simulink model "q_srv02_pos"  (Simulink 6.6)
settings: Solver=ode1  StartTime=0.0  StopTime=inf  FixedStep=0.001  RelTol=1e-3  AbsTol=1e-6
values from neighbouring files (symbols this model uses):
  K_AMP = 1    [setup_srv02_exp02_pos.m]
  ki = -( -AmpMax + kp * e_ss ) / ti / e_ss    [d_i_design.m]    (also in setup_srv02_exp02_pos.m = 0)
  kp = wn^2/K*tau    [d_pv_design.m]    (also in setup_srv02_exp02_pos.m = 0)
  kv = (-1+2*zeta*wn*tau)/K    [d_pv_design.m]    (also in setup_srv02_exp02_pos.m = 0)
  VMAX_DAC = 10    [setup_srv02_exp02_pos.m]
  wcf = 2 * pi * 50.0    (= 314.159265359)    [setup_srv02_exp02_pos.m]
  wcf_e = 2 * pi * 50.0    (= 314.159265359)    [setup_srv02_exp02_pos.m]
  zetaf = 0.9    [setup_srv02_exp02_pos.m]
  zetaf_e = 0.9    [setup_srv02_exp02_pos.m]
undefined symbols (not defined in the file or in its folder): HIL, K_ENC, K_POT, K_TACH, qc_get_step_size, VMAX_AMP
libraries: quarc_library x6
settings Model: Creator=MLevis  LastModifiedBy=MLevis  SimulationMode=external  ExtModeTrigDuration=10000  BufferReuse=off
settings SolverCC: PositivePriorityOrder=on
settings DataIOCC: LimitDataPoints=off
settings OptimizationCC: BlockReduction=off  BooleanDataType=off  InlineInvariantSignals=on  OptimizeBlockIOStorage=off  BufferReuse=off  ExpressionFolding=off  LocalBlockOutputs=off
settings DebuggingCC: SignalResolutionControl=TryResolveAllWithWarning  SolverPrmCheckMsg=none  MultiTaskDSMMsg=warning  MultiTaskCondExecSysMsg=none  StrictBusMsg=None
settings HardwareCC: TargetHWDeviceType=32-bit Generic
settings RTWCC: SystemTargetFile=quarc_windows.tlc  TemplateMakefile=quarc_default_tmf  Description=Quarc Win32 Target  ProcessScript=quarc_windows_make_rtw_hook  IncludeERTFirstTime=on
settings STFCustomTargetCC: TargetFcnLib=ansi_tfl_tmw.mat  TargetPreCompLibLocation=C:\DOCUME~1\ALLUSE~1\APPLIC~1\QUARC\lib\2007a\windows\release  GenFloatMathFcnCalls=ANSI_C  SystemTargetFile=quarc_windows.tlc
settings GRTTargetCC: TargetPreCompLibLocation=C:\DOCUME~1\ALLUSE~1\APPLIC~1\QUARC\lib\2007a\windows\release  MatFileLogging=off  ExtMode=on  ExtModeMexFile=quarc_comm

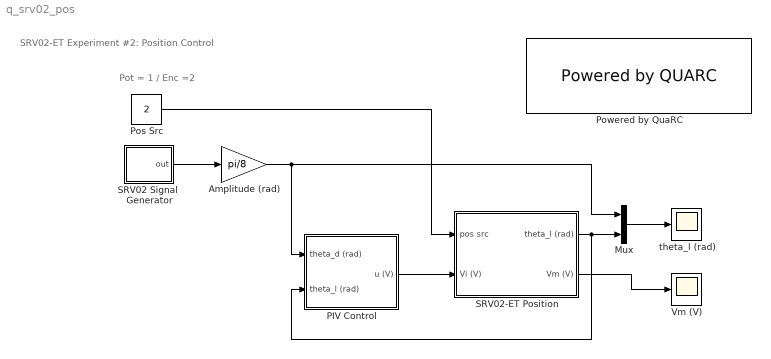
== system q_srv02_pos ==
  note: SRV02-ET Experiment #2: Position Control
  note: Pot = 1 / Enc =2
  Amplitude (rad) : Gain  Gain=pi/8  SaturateOnIntegerOverflow=on
  Mux : Mux  Inputs=2
  PIV Control : Subsystem
  Pos Src : Constant  Value=2
  Powered by QuaRC : quarc_library/Logos/Powered by QUARC  SystemSampleTime=-1
  SRV02 Signal  Generator : Subsystem  mask(QET Signal Generator){sig_type=square, a=1, f=0.4}
      mask prompts: sig_type "Signal Type"; a "Amplitude"; f "Frequency (Hz)"
      mask help: Generates a square, triangular, or sinusoidal waveform of a specified amplitude and frequency.
      mask Help: Choose the type of signal to be generated from the drop-down "Signal Type" box. Enter the amplitude and the frequency desired for the signal. Note: frequency is in Hertz.
      mask StyleString: popup(square|triangle|sine),edit,edit
      mask Display: plot([0 1 1 2 2 3 4 5 6], [-1 -1 1 1 -1 -1 1 -1 -1])
  SRV02-ET Position : Subsystem
  Vm (V) : Scope
      settings: TimeRange=5  YMin=-10  YMax=10  SaveName=data_vm  DataFormat=Array
  theta_l (rad) : Scope
      settings: TimeRange=5  YMin=-1  YMax=1  SaveName=data_pos  DataFormat=Array
  wires:
  Amplitude (rad)/1 -> Mux/1, PIV Control/1(theta_d (rad))
  SRV02-ET Position/1(theta_l (rad)) -> Mux/2, PIV Control/2(theta_l (rad))
  SRV02-ET Position/2(Vm (V)) -> Vm (V)/1
  Mux/1 -> theta_l (rad)/1
  PIV Control/1(u (V)) -> SRV02-ET Position/2(Vi (V))
  SRV02 Signal  Generator/1(out) -> Amplitude (rad)/1
  Pos Src/1 -> SRV02-ET Position/1(pos src)

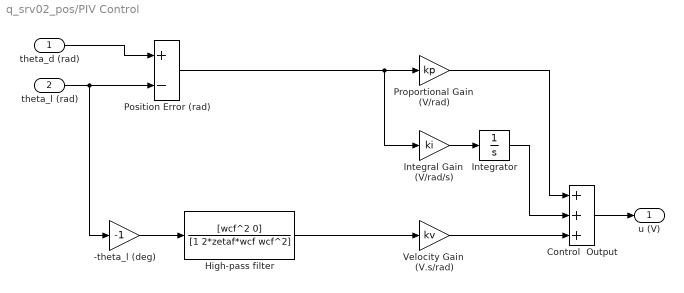
== system q_srv02_pos/PIV Control ==
  theta_d (rad) : Inport
  theta_l (rad) : Inport  Port=2
  -theta_l (deg) : Gain  Gain=-1
  Control  Output : Sum  Inputs=+++  OutScaling=2^-10
  High-pass filter : TransferFcn  Numerator=[wcf^2 0]  Denominator=[1 2*zetaf*wcf wcf^2]
  Integral Gain  (V/rad/s) : Gain  Gain=ki
  Integrator : Integrator  LimitOutput=on  UpperSaturationLimit=VMAX_DAC  LowerSaturationLimit=-VMAX_DAC
  Position Error (rad) : Sum  Inputs=+-  OutScaling=2^-10
  Proportional Gain  (V/rad) : Gain  Gain=kp
  Velocity Gain  (V.s/rad) : Gain  Gain=kv
  u (V) : Outport
  wires:
  Integrator/1 -> Control  Output/2
  Velocity Gain  (V.s/rad)/1 -> Control  Output/3
  Integral Gain  (V/rad/s)/1 -> Integrator/1
  -theta_l (deg)/1 -> High-pass filter/1
  Position Error (rad)/1 -> Proportional Gain  (V/rad)/1, Integral Gain  (V/rad/s)/1
  theta_l (rad)/1 -> -theta_l (deg)/1, Position Error (rad)/2
  Control  Output/1 -> u (V)/1
  theta_d (rad)/1 -> Position Error (rad)/1
  Proportional Gain  (V/rad)/1 -> Control  Output/1
  High-pass filter/1 -> Velocity Gain  (V.s/rad)/1

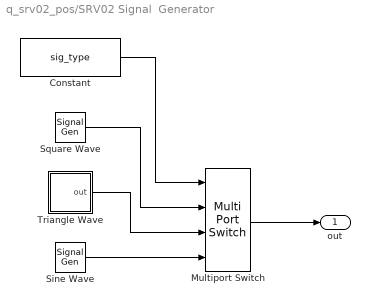
== system q_srv02_pos/SRV02 Signal  Generator ==
  Constant : Constant  Value=sig_type
  Multiport Switch : MultiPortSwitch  Inputs=3
  Sine Wave : SignalGenerator  Amplitude=a  Frequency=f
  Square Wave : SignalGenerator  WaveForm=square  Amplitude=a  Frequency=f
  Triangle Wave : Subsystem
  out : Outport
  wires:
  Constant/1 -> Multiport Switch/1
  Multiport Switch/1 -> out/1
  Sine Wave/1 -> Multiport Switch/4
  Triangle Wave/1(out) -> Multiport Switch/3
  Square Wave/1 -> Multiport Switch/2

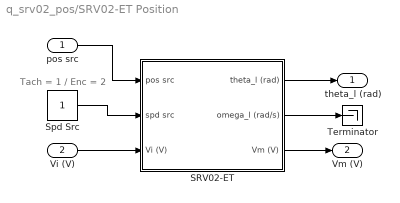
== system q_srv02_pos/SRV02-ET Position ==
  note: Tach = 1 / Enc = 2
  pos src : Inport
  Vi (V) : Inport  Port=2
  SRV02-ET : Subsystem
  Spd Src : Constant
  Terminator : Terminator
  theta_l (rad) : Outport
  Vm (V) : Outport  Port=2
  wires:
  SRV02-ET/2(omega_l (rad/s)) -> Terminator/1
  Spd Src/1 -> SRV02-ET/2(spd src)
  pos src/1 -> SRV02-ET/1(pos src)
  SRV02-ET/1(theta_l (rad)) -> theta_l (rad)/1
  Vi (V)/1 -> SRV02-ET/3(Vi (V))
  SRV02-ET/3(Vm (V)) -> Vm (V)/1

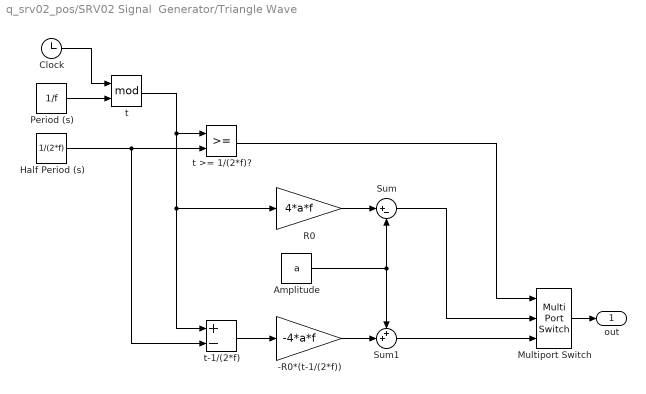
== system q_srv02_pos/SRV02 Signal  Generator/Triangle Wave ==
  -R0*(t-1/(2*f)) : Gain  Gain=-4*a*f
  Amplitude : Constant  Value=a
  Clock : Clock
      settings: Decimation=10
  Half Period (s) : Constant  Value=1/(2*f)
  Multiport Switch : MultiPortSwitch  Inputs=2  zeroidx=on
  Period (s) : Constant  Value=1/f
  R0 : Gain  Gain=4*a*f
  Sum : Sum  Inputs=|+-
  Sum1 : Sum  Inputs=++|
  t : Math  Operator=mod  SaturateOnIntegerOverflow=on
  t >= 1/(2*f)? : RelationalOperator  LogicOutDataTypeMode=Boolean
  t-1/(2*f) : Sum  Inputs=+-  OutScaling=2^-10
  out : Outport
  wires:
  Multiport Switch/1 -> out/1
  Clock/1 -> t/1
  Period (s)/1 -> t/2
  t/1 -> t >= 1/(2*f)?/1, R0/1, t-1/(2*f)/1
  Half Period (s)/1 -> t >= 1/(2*f)?/2, t-1/(2*f)/2
  t-1/(2*f)/1 -> -R0*(t-1/(2*f))/1
  R0/1 -> Sum/1
  Amplitude/1 -> Sum/2, Sum1/1
  -R0*(t-1/(2*f))/1 -> Sum1/2
  t >= 1/(2*f)?/1 -> Multiport Switch/1
  Sum/1 -> Multiport Switch/2
  Sum1/1 -> Multiport Switch/3

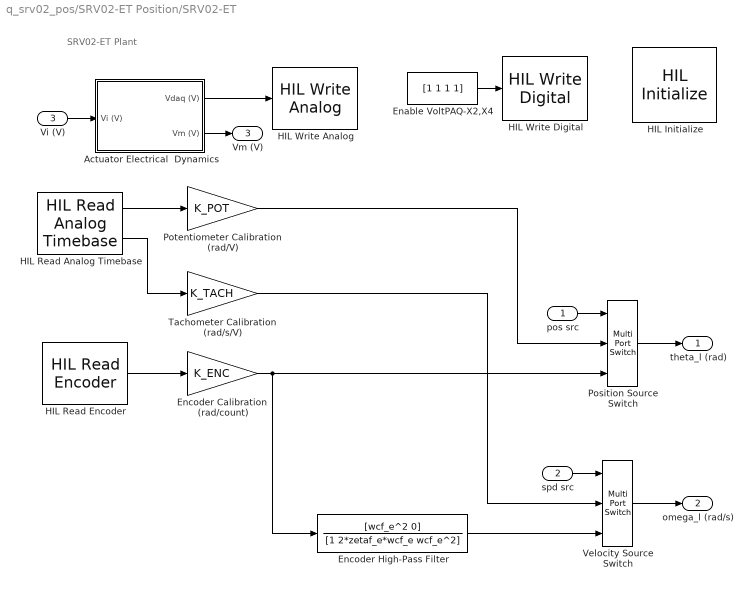
== system q_srv02_pos/SRV02-ET Position/SRV02-ET ==
  note: SRV02-ET Plant
  pos src : Inport
  spd src : Inport  Port=2
  Vi (V) : Inport  Port=3
  Actuator Electrical  Dynamics : Subsystem
  Enable VoltPAQ-X2,X4 : Constant  Value=[1 1 1 1]
  Encoder Calibration  (rad/count) : Gain  Gain=K_ENC  SaturateOnIntegerOverflow=on
  Encoder High-Pass Filter : TransferFcn  Numerator=[wcf_e^2 0]  Denominator=[1 2*zetaf_e*wcf_e wcf_e^2]
  HIL Initialize : quarc_library/Data Acquisition/Generic/Configuration/HIL Initialize  object_name=HIL-1  board_type=q8  board_number=0  exclusive=off  active=off  hardware_clocks=[0:1]  clock_modes=[0 0]  initial_clock_frequencies=[]  set_clock_params_at_start=on  set_clock_params_at_switch_in=off  set_clock_frequencies_at_start=off  set_clock_frequencies_at_switch_in=off  analog_input_channels=[0:7]  analog_input_maximums=10  analog_input_minimums=-10  set_analog_input_params_at_start=off  set_analog_input_params_at_switch_in=off  analog_output_channels=[0:7]  analog_output_maximums=[10]  analog_output_minimums=[-10]  initial_analog_outputs=[0]  final_analog_outputs=[0]  watchdog_analog_outputs=0  set_analog_output_params_at_start=on  set_analog_output_params_at_switch_in=off  set_analog_outputs_at_start=on  set_analog_outputs_at_switch_in=off  set_analog_outputs_at_terminate=on  set_analog_outputs_at_switch_out=off  set_analog_outputs_on_watchdog=on  digital_input_channels=[16:31]  digital_output_channels=[0:15]  digital_output_configuration=[]  initial_digital_outputs=[0]  final_digital_outputs=[0]  watchdog_digital_outputs=[2]  set_digital_output_params_at_start=off  set_digital_output_params_at_switch_in=off  set_digital_outputs_at_start=on  set_digital_outputs_at_switch_in=off  set_digital_outputs_at_terminate=on  set_digital_outputs_at_switch_out=off  set_digital_outputs_on_watchdog=off  encoder_channels=[0:7]  quadrature=[4]  encoder_filter_frequency=(1/120e-9)/1  initial_encoder_counts=[0]  set_encoder_params_at_start=on  set_encoder_params_at_switch_in=off  set_encoder_counts_at_start=on  set_encoder_counts_at_switch_in=off  pwm_channels=[]  pwm_modes=[0]  pwm_frequency=(1/60e-9)/1024  pwm_configuration=[]  pwm_alignment=[]  pwm_polarity=[]  pwm_leading_deadband=[]  pwm_trailing_deadband=[]  initial_pwm_outputs=[0]  final_pwm_outputs=[0]  watchdog_pwm_outputs=[]  set_pwm_params_at_start=on  set_pwm_params_at_switch_in=off  set_pwm_outputs_at_start=on  set_pwm_outputs_at_switch_in=off  set_pwm_outputs_at_terminate=on  set_pwm_outputs_at_switch_out=off  set_pwm_outputs_on_watchdog=off  other_output_channels=[]  initial_other_outputs=[]  final_other_outputs=[]  watchdog_other_outputs=[]  set_other_outputs_at_start=off  set_other_outputs_at_switch_in=off  set_other_outputs_at_terminate=off  set_other_outputs_at_switch_out=off  set_other_outputs_on_watchdog=off
  HIL Read Analog Timebase : quarc_library/Data Acquisition/Generic/Timebases/HIL Read Analog Timebase  Tag=unassigned  object_name=HIL-1  clock=0  channels=[0:1]  samples_in_buffer=max(ceil(1/qc_get_step_size), 1)  active=on  vector_output=off
      settings: AttributesFormatString=(%<object_name>)
  HIL Read Encoder : quarc_library/Data Acquisition/Generic/Immediate I//O/HIL Read Encoder  Tag=unassigned  object_name=HIL-1  channels=0  sample_time=qc_get_step_size  active=on  vector_output=off  data_type_mode=Inherit via back propagation  data_type=double
  HIL Write Analog : quarc_library/Data Acquisition/Generic/Immediate I//O/HIL Write Analog  Tag=unassigned  object_name=HIL-1  channels=0  sample_time=-1  active=off  vector_input=off
  HIL Write Digital : quarc_library/Data Acquisition/Generic/Immediate I//O/HIL Write Digital  object_name=HIL-1  channels=[0:3]  sample_time=-1  active=off  vector_input=on
  Position Source Switch : MultiPortSwitch  Inputs=2
  Potentiometer Calibration  (rad/V) : Gain  Gain=K_POT  SaturateOnIntegerOverflow=on
  Tachometer Calibration  (rad/s/V) : Gain  Gain=K_TACH  SaturateOnIntegerOverflow=on
  Velocity Source Switch : MultiPortSwitch  Inputs=2
  theta_l (rad) : Outport  InitialOutput=0
  omega_l (rad/s) : Outport  Port=2  InitialOutput=0
  Vm (V) : Outport  Port=3  InitialOutput=0
  wires:
  HIL Read Analog Timebase/2 -> Tachometer Calibration  (rad/s/V)/1
  HIL Read Encoder/1 -> Encoder Calibration  (rad/count)/1
  Encoder High-Pass Filter/1 -> Velocity Source Switch/3
  Potentiometer Calibration  (rad/V)/1 -> Position Source Switch/2
  spd src/1 -> Velocity Source Switch/1
  pos src/1 -> Position Source Switch/1
  Position Source Switch/1 -> theta_l (rad)/1
  Velocity Source Switch/1 -> omega_l (rad/s)/1
  HIL Read Analog Timebase/1 -> Potentiometer Calibration  (rad/V)/1
  Vi (V)/1 -> Actuator Electrical  Dynamics/1(Vi (V))
  Encoder Calibration  (rad/count)/1 -> Encoder High-Pass Filter/1, Position Source Switch/3
  Tachometer Calibration  (rad/s/V)/1 -> Velocity Source Switch/2
  Actuator Electrical  Dynamics/1(Vdaq (V)) -> HIL Write Analog/1
  Actuator Electrical  Dynamics/2(Vm (V)) -> Vm (V)/1
  Enable VoltPAQ-X2,X4/1 -> HIL Write Digital/1

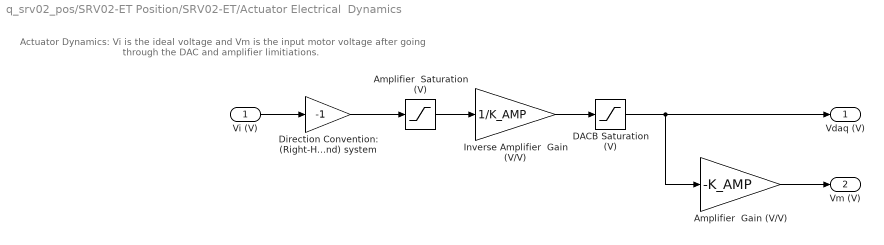
== system q_srv02_pos/SRV02-ET Position/SRV02-ET/Actuator Electrical  Dynamics ==
  note: Actuator Dynamics: Vi is the ideal voltage and Vm is the
      | input motor voltage after going through the DAC and amplifier limitiations.
  Vi (V) : Inport
  Amplifier  Gain (V/V) : Gain  Gain=-K_AMP
  Amplifier  Saturation (V) : Saturate  UpperLimit=VMAX_AMP  LowerLimit=-VMAX_AMP
  DACB Saturation (V) : Saturate  UpperLimit=VMAX_DAC  LowerLimit=-VMAX_DAC
  Direction Convention: (Right-Hand) system : Gain  Gain=-1  SaturateOnIntegerOverflow=on
  Inverse Amplifier  Gain (V/V) : Gain  Gain=1/K_AMP
  Vdaq (V) : Outport
  Vm (V) : Outport  Port=2
  wires:
  Vi (V)/1 -> Direction Convention: (Right-Hand) system/1
  Amplifier  Saturation (V)/1 -> Inverse Amplifier  Gain (V/V)/1
  Inverse Amplifier  Gain (V/V)/1 -> DACB Saturation (V)/1
  DACB Saturation (V)/1 -> Amplifier  Gain (V/V)/1, Vdaq (V)/1
  Amplifier  Gain (V/V)/1 -> Vm (V)/1
  Direction Convention: (Right-Hand) system/1 -> Amplifier  Saturation (V)/1
